simulink model "diagrama4"  (Simulink 9.1)
settings: Solver=VariableStepAuto  StartTime=0.0  StopTime=20  RelTol=1e-3  EnableMultiTasking=on
undefined symbols (not defined in the file or in its folder): Fs
libraries: dspobslib x7, dspsigops x1, dspsrcs4 x1, dspstat3 x1
settings Model: Creator=tcom00  LastModifiedBy=Eduardo  ExtModeAutoUpdateStatusClock=off
settings DataIOCC: LimitDataPoints=on  SignalLoggingSaveFormat=ModelDataLogs  SignalLoggingName=sigsOut
settings OptimizationCC: ExpressionDepthLimit=2147483647
settings DebuggingCC: SaveWithParameterizedLinksMsg=none  SignalResolutionControl=TryResolveAllWithWarning  MultiTaskDSMMsg=warning  MultiTaskCondExecSysMsg=none  FcnCallInpInsideContextMsg=warning  AllowSymbolicDim=off  StateNameClashWarn=warning
settings HardwareCC: TargetUnknown=on
settings GRTTargetCC: GeneratePreprocessorConditionals=Disable all

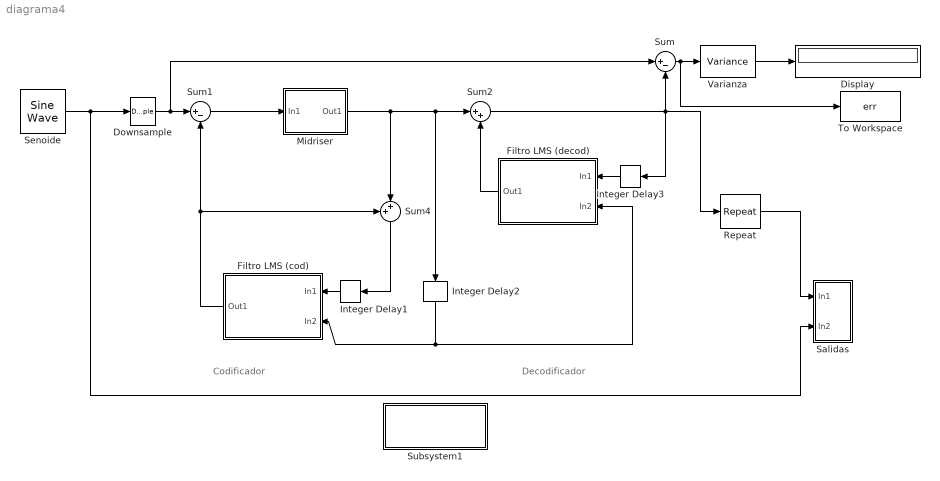
== system diagrama4 ==
  note: Codificador
  note: Decodificador
  Display : Display
  Downsample : DownSample  N=4  InputProcessing=Inherited (this choice will be removed - see release notes)  RateOptions=Allow multirate processing
  Filtro LMS (cod) : Subsystem
      mask Display:
      | disp('LMS');
      | port_label('input', 1, 'In');
      | port_label('input', 2, 'Err');
      | port_label('output', 1, 'Out');
  Filtro LMS (decod) : Subsystem
      mask Display:
      | disp('LMS');
      | port_label('input', 1, 'In');
      | port_label('input', 2, 'Err');
      | port_label('output', 1, 'Out');
  Integer Delay1 : dspobslib/Integer Delay  delay=1  ic=0  reset_popup=None
      settings: SourceProductName=DSP System Toolbox  SourceProductBaseCode=DS
  Integer Delay2 : dspobslib/Integer Delay  delay=1  ic=0  reset_popup=None
      settings: SourceProductName=DSP System Toolbox  SourceProductBaseCode=DS
  Integer Delay3 : dspobslib/Integer Delay  delay=1  ic=0  reset_popup=None
      settings: SourceProductName=DSP System Toolbox  SourceProductBaseCode=DS
  Midriser : Subsystem  mask{L=16, xsc=1}
      mask prompts: L "niveles"
      mask Display: image('.\png\midriser.png');
  Repeat : dspsigops/Repeat  N=4  InputProcessing=Columns as channels (frame based)  RateOptions=Allow multirate processing  ic=0  mode=Unused parameter value
      settings: SourceProductName=DSP System Toolbox
  Salidas : Subsystem
      mask Display:
      | plot([0, 1], [1, 1]);
      | plot([0, 0], [1, 0.5]);
      | plot([0, 1], [0.5, 0.5]);
      | plot([1, 1], [1, 0.5]);
      | disp('\n\nMulti\nscope');
  Senoide : dspsrcs4/Sine Wave  Amplitude=1  Frequency=1000  Phase=0  SampleMode=Discrete  OutComplex=Real  CompMethod=Trigonometric fcn  TableSize=Speed  SampleTime=1/200000  SamplesPerFrame=1  ResetState=Restart at time zero  OutputFrames=on  dataType=double  wordLen=16  udDataType=sfix(16)  fracBitsMode=Best precision  numFracBits=14  OutDataTypeStr=double  LastOutDataTypeStr=double
  Subsystem1 : Subsystem  mask{L=16, xsc=1}
      mask prompts: L "Niveles :"; xsc "xsc :"
      mask Callback L:
      | L = get_param(gcb, 'L');
      | set_param([bdroot '/Midriser'], 'L',L);
      mask Callback xsc:
      | xsc = get_param(gcb, 'xsc');
      | set_param([bdroot '/Midriser'], 'xsc',xsc);
      mask Display: disp('Parametros del\nsistema');
  Sum : Sum  Inputs=|+-  SaturateOnIntegerOverflow=on
  Sum1 : Sum  Inputs=|+-  SaturateOnIntegerOverflow=on
  Sum2 : Sum  Inputs=|++  SaturateOnIntegerOverflow=on
  Sum4 : Sum  Inputs=++|  SaturateOnIntegerOverflow=on
  To Workspace : ToWorkspace  VariableName=err  SampleTime=-1
      settings: Save2DSignal=2-D array (concatenate along first dimension)
  Varianza : dspstat3/Variance  run=on  InputProcessing=Columns as channels (frame based)  reset_popup=None  directionMode=Each column  dimension=1  roiEnable=off  roiType=Rectangles  roiPortion=Entire ROI  roiOutput=Individual statistics for each ROI  roiFlag=off  roundingMode=Floor  overflowMode=off
      settings: SourceProductName=DSP System Toolbox
  wires:
  Senoide/1 -> Downsample/1, Salidas/2(In2)
  Filtro LMS (cod)/1(Out1) -> Sum1/2, Sum4/1
  Sum4/1 -> Integer Delay1/1
  Integer Delay1/1 -> Filtro LMS (cod)/1(In1)
  Filtro LMS (decod)/1(Out1) -> Sum2/2
  Sum2/1 -> Repeat/1, Integer Delay3/1, Sum/2
  Sum/1 -> Varianza/1, To Workspace/1
  Integer Delay3/1 -> Filtro LMS (decod)/1(In1)
  Integer Delay2/1 -> Filtro LMS (cod)/2(In2), Filtro LMS (decod)/2(In2)
  Varianza/1 -> Display/1
  Repeat/1 -> Salidas/1(In1)
  Downsample/1 -> Sum1/1, Sum/1
  Sum1/1 -> Midriser/1(In1)
  Midriser/1(Out1) -> Integer Delay2/1, Sum2/1, Sum4/2

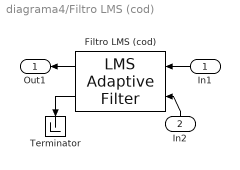
== system diagrama4/Filtro LMS (cod) ==
  In1 : Inport
  In2 : Inport  Port=2
  Filtro LMS (cod) : dspobslib/LMS Adaptive Filter  n=16  mu=1e-5  ic=[1, zeros(1, 15)]'  leakage=1  normalized=off  Adapt=off  RstPort=None
      settings: SourceProductName=DSP System Toolbox  SourceProductBaseCode=DS
  Terminator : Terminator
  Out1 : Outport
  wires:
  Filtro LMS (cod)/2 -> Terminator/1
  In2/1 -> Filtro LMS (cod)/2
  In1/1 -> Filtro LMS (cod)/1
  Filtro LMS (cod)/1 -> Out1/1

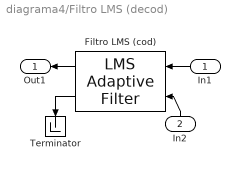
== system diagrama4/Filtro LMS (decod) ==
  In1 : Inport
  In2 : Inport  Port=2
  Filtro LMS (cod) : dspobslib/LMS Adaptive Filter  n=16  mu=1e-5  ic=[1, zeros(1, 15)]'  leakage=1  normalized=off  Adapt=off  RstPort=None
      settings: SourceProductName=DSP System Toolbox  SourceProductBaseCode=DS
  Terminator : Terminator
  Out1 : Outport
  wires:
  Filtro LMS (cod)/2 -> Terminator/1
  In2/1 -> Filtro LMS (cod)/2
  In1/1 -> Filtro LMS (cod)/1
  Filtro LMS (cod)/1 -> Out1/1

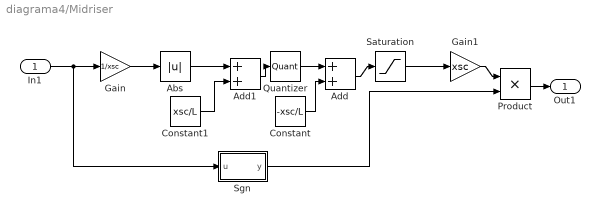
== system diagrama4/Midriser ==
  In1 : Inport
  Abs : Abs
  Add : Sum
  Add1 : Sum
  Constant : Constant  Value=-xsc/L
  Constant1 : Constant  Value=xsc/L
  Gain : Gain  Gain=1/xsc
  Gain1 : Gain  Gain=xsc
  Product : Product
  Quantizer : Quantizer  QuantizationInterval=2*xsc/L
  Saturation : Saturate  UpperLimit=xsc-xsc/L  LowerLimit=-xsc+xsc/L
  Sgn : MATLAB Function  TreatAsAtomicUnit=on
  Out1 : Outport
  wires:
  In1/1 -> Gain/1, Sgn/1(u)
  Product/1 -> Out1/1
  Quantizer/1 -> Add/1
  Sgn/1(y) -> Product/2
  Constant/1 -> Add/2
  Add/1 -> Saturation/1
  Gain1/1 -> Product/1
  Saturation/1 -> Gain1/1
  Add1/1 -> Quantizer/1
  Gain/1 -> Abs/1
  Constant1/1 -> Add1/2
  Abs/1 -> Add1/1

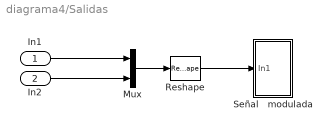
== system diagrama4/Salidas ==
  In1 : Inport
  In2 : Inport  Port=2
  Mux : Mux  Inputs=2
  Reshape : Reshape  OutputDimensionality=Row vector (2-D)
  Señal   modulada : Subsystem
      mask Display:
      | plot([0, 1], [1, 1]);
      | plot([0, 0], [1, 0.5]);
      | plot([0, 1], [0.5, 0.5]);
      | plot([1, 1], [1, 0.5]);
      | disp('\n\nFrame\nscope');
  wires:
  Mux/1 -> Reshape/1
  Reshape/1 -> Señal   modulada/1(In1)
  In1/1 -> Mux/1
  In2/1 -> Mux/2

== system diagrama4/Subsystem1 ==

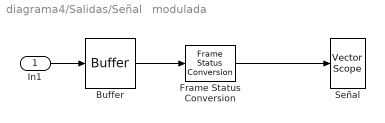
== system diagrama4/Salidas/Señal   modulada ==
  In1 : Inport
  Buffer : Buffer  N=400
  Frame Status Conversion : dspobslib/Frame Status Conversion  growRefPort=off  outframe=Frame-based
      settings: SourceProductName=DSP System Toolbox  SourceProductBaseCode=DS
  Señal : dspobslib/Vector Scope  ScopeProperties=on  Domain=User-defined  HorizSpan=1  DisplayProperties=off  AxisGrid=on  Memory=off  FrameNumber=off  AxisLegend=off  AxisZoom=off  OpenScopeAtSimStart=on  OpenScopeImmediately=off  FigPos=[512, 50, 512, 300]  AxisProperties=off  XUnits=rad/sec  XRange=[-Fs/2...Fs/2]  InheritXIncr=on  XIncr=1  XLabel=Tiempo (s)  XLimit=Auto  XMin=0  XMax=1  XStart=0  YUnits=Magnitude  YLabel=Amplitud  LineProperties=off  LineColors='b' | 'r'  XAxisParamsVer=6.8
      settings: SourceProductName=DSP System Toolbox  SourceProductBaseCode=DS  YMin=-1.09998180162849  YMax=1.10498171890862
  wires:
  Buffer/1 -> Frame Status Conversion/1
  Frame Status Conversion/1 -> Señal/1
  In1/1 -> Buffer/1

== matlab function Midriser/Sgn ==
  data: u input double; y output double
function y = fcn(u)

if u~=0
    y=sign(u);
else
    y=1;
end
